simulink model "Convert_Frame_Scalar"  (R2018a)
settings: Solver=VariableStepAuto  StartTime=0.0  StopTime=10.0  RelTol=1e-3
libraries: dspsrcs4 x1
settings Model: Creator=hpong  LastModifiedBy=hpong

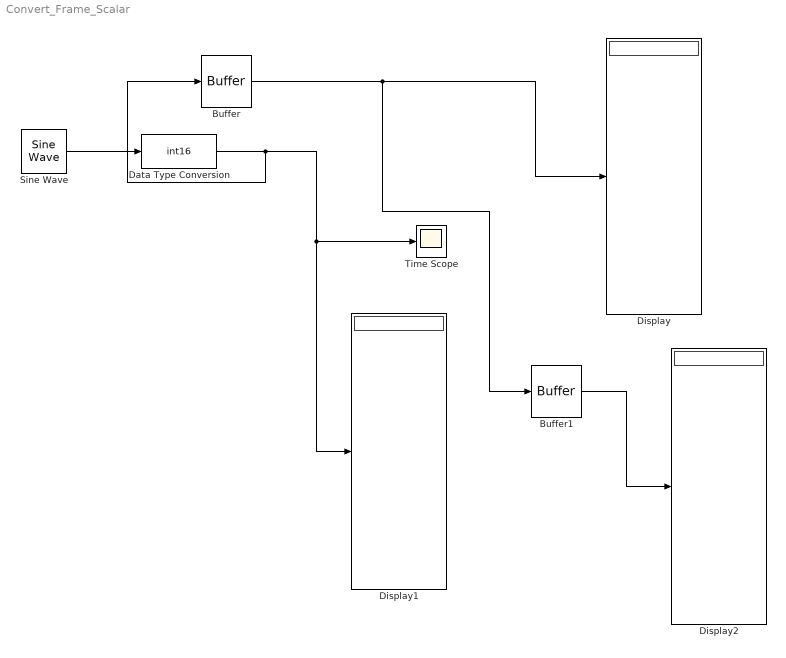
== system Convert_Frame_Scalar ==
  Buffer : Buffer  N=1  OutputFrames=off
  Buffer1 : Buffer  N=12  OutputFrames=off
  Data Type Conversion : DataTypeConversion  OutDataTypeStr=int16
  Display : Display
  Display1 : Display
  Display2 : Display
  Sine Wave : dspsrcs4/Sine Wave  Amplitude=32768  Frequency=1000  Phase=0  SampleMode=Discrete  OutComplex=Real  CompMethod=Trigonometric fcn  TableSize=Speed  SampleTime=1/48000  SamplesPerFrame=12  ResetState=Restart at time zero  OutputFrames=off  dataType=single  wordLen=16  udDataType=sfix(16)  fracBitsMode=Best precision  numFracBits=15  OutDataTypeStr=single  LastOutDataTypeStr=single
  Time Scope : Scope
  wires:
  Sine Wave/1 -> Data Type Conversion/1
  Buffer/1 -> Buffer1/1, Display/1
  Data Type Conversion/1 -> Buffer/1, Display1/1, Time Scope/1
  Buffer1/1 -> Display2/1
